simulink model "ctrl_DPAD_2"  (R2016b)
settings: Solver=ode3  StartTime=0.0  StopTime=inf  FixedStep=0.01  RelTol=1e-3  EnableMultiTasking=on
values from neighbouring files (symbols this model uses):
  C = [C1;C2;C3;C4;C5;C6]    [initfile.m]
  D = 3.0/100    (= 0.03)    [initfile.m]
  eps_c = 5    [initfile.m]
  epsilon = 0.5    [initfile.m]
  hd = c2d(H1,0.01,'foh')    [initfile.m]
  hd2 = c2d(H2,0.01,'zoh')    [initfile.m]
  I_s = 25000 /747225    (= 0.0334571246947)    [initfile.m]
  k_cc = 1    [initfile.m]
  K_omega = 0.3    [initfile.m]
  K_q1f = 0.0113    [initfile.m]
  K_q1r = K_q1f    (= 0.0113)    [initfile.m]
  K_q2f = 0.0117    [initfile.m]
  K_q2r = K_q2f    (= 0.0117)    [initfile.m]
  K_q3f = 0.0113    [initfile.m]
  K_q3r = K_q3f    (= 0.0113)    [initfile.m]
  K_q4f = 0.0169    [initfile.m]
  K_q4r = K_q4f    (= 0.0169)    [initfile.m]
  K_q5f = 0.0144    [initfile.m]
  K_q5r = K_q5f    (= 0.0144)    [initfile.m]
  K_q6f = 0.0168    [initfile.m]
  K_q6r = K_q6f    (= 0.0168)    [initfile.m]
  K_T1f = 0.3763    [initfile.m]
  K_T1r = K_T1f    (= 0.3763)    [initfile.m]
  K_T2f = 0.3901    [initfile.m]
  K_T2r = K_T2f    (= 0.3901)    [initfile.m]
  K_T3f = 0.3776    [initfile.m]
  K_T3r = K_T3f    (= 0.3776)    [initfile.m]
  K_T4f = 0.5641    [initfile.m]
  K_T4r = K_T4f    (= 0.5641)    [initfile.m]
  K_T5f = 0.4799    [initfile.m]
  K_T5r = K_T5f    (= 0.4799)    [initfile.m]
  K_T6f = 0.5588    [initfile.m]
  K_T6r = K_T6f    (= 0.5588)    [initfile.m]
  Kp = 3.3    [initfile.m]
  Max_Acceleration = 5    [initfile.m]
  Max_rotation = 12*sqrt(lambda)    [initfile.m]
  Max_thrust = 1.5    [initfile.m]
  Min_thrust = -0.8    [initfile.m]
  n_c = 5    [initfile.m]
  n_max = 152    [initfile.m]
  p_cc = 0.5    [initfile.m]
  pwm_thr1_backward = coeffvalues(ForceToPWM)    [initfile.m]
  pwm_thr1_forward = coeffvalues(ForceToPWM)    [initfile.m]
  pwm_thr2_backward = coeffvalues(ForceToPWM)    [initfile.m]
  pwm_thr2_forward = coeffvalues(ForceToPWM)    [initfile.m]
  pwm_thr3_backward = coeffvalues(ForceToPWM)    [initfile.m]
  pwm_thr3_forward = coeffvalues(ForceToPWM)    [initfile.m]
  pwm_thr4_backward = coeffvalues(ForceToPWM)    [initfile.m]
  pwm_thr4_forward = coeffvalues(ForceToPWM)    [initfile.m]
  pwm_thr5_backward = coeffvalues(ForceToPWM)    [initfile.m]
  pwm_thr5_forward = coeffvalues(ForceToPWM)    [initfile.m]
  pwm_thr6_backward = coeffvalues(ForceToPWM)    [initfile.m]
  pwm_thr6_forward = coeffvalues(ForceToPWM)    [initfile.m]
  Q_f0 = 0.3    [initfile.m]
  r_cc = 4    [initfile.m]
  Rho = Rho_m    (= 1000)    [initfile.m]
undefined symbols (not defined in the file or in its folder): DiscIntNeverNeededParam, Q_max, Thruster
libraries: marine_gnc x8, simulink x6, simulink_extras x3
(part 5 of 5)

== matlab function ctrl_DPAD_2/Thrust allocation/MATLAB Function ==
  data: u input; sys output; ThrusterPosX input; ThrusterPosY input; C input
function sys = fcn(u,ThrusterPosX,ThrusterPosY,C)
% Complete system goes here!
Alpha1 = zeros(1,6);    % Allocating dimensions for faster computing
% Parameters thrusters
tc =  [u(1),u(2),u(3)]'; 
alpha = [u(4),u(5),u(6),u(7),u(8),u(9)]';

% Constraints for Thruster-Thruster interaction. Can be seen in "Initfile"
% how they are found
C1 = C(1,:);
C2 = C(2,:);
C3 = C(3,:);
C4 = C(4,:);
C5 = C(5,:);
C6 = C(6,:);

K = ones(1,6);

K = ones(1,6);

if alpha(1) < C1(1)-0.1  && alpha(1) > C1(2)+0.1 || alpha(1) > C1(3)+0.1 && alpha(1) < C1(4)-0.1
    K(1) = 0;
else 
    K(1) = K(1);
end

if alpha(2) > C2(1)-0.1  && alpha(2) < C2(2)+0.1 || alpha(2) > C2(3)-0.1 && alpha(2) < C2(4)+0.1
    K(2) = 0;
else 
    K(2) = K(2);
end

if alpha(3) < C3(1)+0.1  && alpha(3) > C3(2)-0.1 || alpha(3) < C3(3)+0.1 && alpha(3) > C3(4)-0.1
    K(3) = 0;
else 
    K(3) = K(3);
end

if alpha(4) > C4(1)+0.1  && alpha(4) < C4(2)-0.1 || alpha(4) < C4(3)-0.1 && alpha(4) > C4(4)+0.1
    K(4) = 0;
else 
    K(4) = K(4);
end

if alpha(5) < C5(1)-0.1  && alpha(5) > C5(2)+0.1 || alpha(5) < C5(3)-0.1 && alpha(5) > C5(4)+0.1
    K(5) = 0;
else 
    K(5) = K(5);
end

if alpha(6) > C6(1)+0.1  && alpha(6) < C6(2)-0.1 || alpha(6) > C6(3)+0.1 && alpha(6) < C6(4)-0.1
    K(6) = 0;
else 
    K(6) = K(6);
end

epsilon = u(10);

n_t = length(ThrusterPosX); % number of thrusters
B_surge = zeros(n_t,1); % Shells for faster computing
B_sway = zeros(n_t,1);  % Shells for faster computing
B_yaw = zeros(n_t,1);   % Shells for faster computing

for i = 1:1:n_t
  B_surge(i) = cosd(alpha(i));     %Thrust in x-direction for cartesian
  B_sway(i) = sind(alpha(i));      %Thrust in y-direction for cartesian
  B_yaw(i) = (sind(alpha(i))*ThrusterPosX(i) - cosd(alpha(i))*ThrusterPosY(i));
end


B = [B_surge,B_sway,B_yaw]';
B = B*diag(K); 
[U_singular,S_singular,V_singular] = svd(B,'econ');
S_singular_cross = 1./S_singular;
S_singular_cross(~isfinite(S_singular_cross))=0;
 if (S_singular_cross(3,3)>10*S_singular_cross(2,2)) 
     S_singular_cross(3,3)=0;
 end
 
u_optimized = V_singular*S_singular_cross*U_singular';

u_d = u_optimized*tc;          % Optimized Thrust



Te = [1 0 1 0 1 0 1 0 1 0 1 0;
      0 1 0 1 0 1 0 1 0 1 0 1;
      ThrusterPosY(1) ThrusterPosX(1) ThrusterPosY(2) ThrusterPosX(2) ThrusterPosY(3) ThrusterPosX(3) ...
      ThrusterPosY(4) ThrusterPosX(4) ThrusterPosY(5) ThrusterPosX(5) ThrusterPosY(6) ThrusterPosX(6)];

[U_singular,S_singular,V_singular] = svd(Te,'econ');
S_singular_cross = 1./S_singular;
S_singular_cross(~isfinite(S_singular_cross))=0;
 if (S_singular_cross(3,3)>2*S_singular_cross(2,2)) 
     S_singular_cross(3,3)=0;
 end
T0 = V_singular*S_singular_cross*U_singular'*tc;

alpha1 = [atan2d(T0(2),T0(1)) atan2d(T0(4),T0(3)) atan2d(T0(6),T0(5)) atan2d(T0(8),T0(7)) atan2d(T0(10),T0(9)) atan2d(T0(12),T0(11))];


%% Constraints
% Thruster 1 OK
%C1 = [151 130 -151 -130 ];
if alpha1(1) < C1(1)  && alpha1(1) > C1(2) && u_d(1) > 0 || alpha1(1) < C1(1)  && alpha1(1) > C1(2) && u_d(1) < 0
    c1 = [C1(1) C1(2)];
    [C_1,alpha_new1] = min(abs(c1-alpha1(1)));
    Alpha1(1) = c1(alpha_new1);
elseif alpha1(1) > C1(3) && alpha1(1) < C1(4) && u_d(1) > 0 || alpha1(1) > C1(3) && alpha1(1) < C1(4) && u_d(1) < 0
    c1 = [C1(3) C1(4)];
    [C_1,alpha_new1] = min(abs(c1-alpha1(1)));
    Alpha1(1) = c1(alpha_new1);
else 
    Alpha1(1) = alpha1(1);
end
if alpha(1) < C1(1)-0.1  && alpha(1) > C1(2)+0.1 || alpha(1) > C1(3)+0.1 && alpha(1) < C1(4)-0.1
    u_d(1) = 0;
else 
    u_d(1) = u_d(1);
end

% Thruster 2 
%C2 = [-99.85 -80.15 -50 -29];
if alpha1(2) < C2(1)  && alpha1(2) > C2(2) && u_d(2) > 0 || alpha1(2) < C2(1)  && alpha1(2) > C2(2) && u_d(2) < 0 
    c2 = [C2(1) C2(2)];
    [C_2,alpha_new2] = min(abs(c2-alpha1(2)));
    Alpha1(2) = c2(alpha_new2);
elseif alpha1(2) < C2(3) && alpha1(2) > C2(4) && u_d(2) > 0 || alpha1(2) < C2(3) && alpha1(2) > C2(4) && u_d(2) < 0
    c2 = [C2(3) C2(4)];
    [C_2,alpha_new2] = min(abs(c2-alpha1(2)));
    Alpha1(2) = c2(alpha_new2);
else 
    Alpha1(2) = alpha1(2);
end
if alpha(2) < C2(1)-0.1  && alpha(2) > C2(2)+0.1 || alpha(2) < C2(3)-0.1 && alpha(2) > C2(4)+0.1
    u_d(2) = 0;
else 
    u_d(2) = u_d(2);
end

% Thruster 3 
% C3 = [99.85 80.15 50 29]; 

if alpha1(3) > C3(1)  && alpha1(3) < C3(2) && u_d(3) > 0 || alpha1(3) > C3(1)  && alpha1(3) < C3(2) && u_d(3) < 0
    c3 = [C3(1) C3(2)];
    [C_3,alpha_new3] = min(abs(c3-alpha1(3)));
    Alpha1(3) = c3(alpha_new3);
elseif alpha1(3) > C3(3) && alpha1(3) < C3(4) && u_d(3) > 0 || alpha1(3) > C3(3) && alpha1(3) < C3(4) && u_d(3) < 0 
    c3 = [C3(3) C3(4)];
    [C_3,alpha_new3] = min(abs(c3-alpha1(3)));
    Alpha1(3) = c3(alpha_new3);
else 
    Alpha1(3) = alpha1(3);
end
if alpha(3) > C3(1)+0.1  && alpha(3) < C3(2)-0.1 || alpha(3) > C3(3)+0.1 && alpha(3) < C3(4)-0.1
    u_d(3) = 0;
else 
    u_d(3) = u_d(3);
end

% Thruster 4 OK
%C4 = [-52.8 -34.2 52.8 34.2]; 
if alpha1(4) > C4(1)  && alpha1(4) < C4(2) && u_d(4) > 0 || alpha1(4) > C4(1)  && alpha1(4) < C4(2) && u_d(4) < 0
    c4 = [C4(1) C4(2)];
    [C_4,alpha_new4] = min(abs(c4-alpha1(4)));
    Alpha1(4) = c4(alpha_new4);
elseif alpha1(4) < C4(3) && alpha1(4) > C4(4) && u_d(4) > 0 || alpha1(4) < C4(3) && alpha1(4) > C4(4) && u_d(4) < 0 
    c4 = [C4(3) C4(4)];
    [C_4,alpha_new4] = min(abs(c4-alpha1(4)));
    Alpha1(4) = c4(alpha_new4);
else 
    Alpha1(4) = alpha1(4);
end
if alpha(4) > C4(1)+0.1  && alpha(4) < C4(2)-0.1 || alpha(4) < C4(3)-0.1 && alpha(4) > C4(4)+0.1
    u_d(4) = 0;
else 
    u_d(4) = u_d(4);
end

% Thruster 5
%C5 = [-98.25 -81.75 -145.8 -127.2];
if alpha1(5) < C5(1)  && alpha1(5) > C5(2) && u_d(5) > 0 || alpha1(5) < C5(1)  && alpha1(5) > C5(2) && u_d(5) < 0
    c5 = [C5(1) C5(2)];
    [C_5,alpha_new5] = min(abs(c5-alpha1(5)));
    Alpha1(5) = c5(alpha_new5);
elseif alpha1(5) < C5(3) && alpha1(5) > C5(4) && u_d(5) > 0  || alpha1(5) < C5(3) && alpha1(5) > C5(4) && u_d(5) < 0
    c5 = [C5(3) C5(4)];
    [C_5,alpha_new5] = min(abs(c5-alpha1(5)));
    Alpha1(5) = c5(alpha_new5);
else 
    Alpha1(5) = alpha1(5);
end
if alpha(5) < C5(1)-0.1  && alpha(5) > C5(2)+0.1 || alpha(5) < C5(3)-0.1 && alpha(5) > C5(4)+0.1
    u_d(5) = 0;
else 
    u_d(5) = u_d(5);
end

% Thruster 6
%C6 = [98.75 81.75 145.8 127.2];
if alpha1(6) > C6(1)  && alpha1(6) < C6(2) && u_d(6) > 0 || alpha1(6) > C6(1)  && alpha1(6) < C6(2) && u_d(6) < 0
    c6 = [C6(1) C6(2)];
    [C_6,alpha_new6] = min(abs(c6-alpha1(6)));
    Alpha1(6) = c6(alpha_new6);
elseif alpha1(6) > C6(3) && alpha1(6) < C6(4) && u_d(6) > 0 || alpha1(6) > C6(3) && alpha1(6) < C6(4) && u_d(6) < 0
    c6 = [C6(3) C6(4)];
    [C_6,alpha_new6] = min(abs(c6-alpha1(6)));
    Alpha1(6) = c6(alpha_new6);
else 
    Alpha1(6) = alpha1(6);
end
if alpha(6) > C6(1)+0.1  && alpha(6) < C6(2)-0.1 || alpha(6) > C6(3)+0.1 && alpha(6) < C6(4)-0.1
    u_d(6) = 0;
else 
    u_d(6) = u_d(6);
end

% Thruster 2&3 
if Alpha1(2) == C2(2)
    Alpha1(3) = alpha1(2) - (C2(2) - alpha1(2));
elseif Alpha1(2) == C2(1)
    Alpha1(3) = alpha1(2) - (C2(1) - alpha1(2));
elseif Alpha1(2) == C2(3)
    Alpha1(3) = alpha1(2) - (C2(3) - alpha1(2));
elseif Alpha1(2) == C2(4)
    Alpha1(3) = alpha1(2) - (C2(4) - alpha1(2));
    
elseif Alpha1(3) == C3(2)
    Alpha1(2) = alpha1(3) - (C3(2) - alpha1(3));
elseif Alpha1(3) == C3(1)
    Alpha1(2) = alpha1(3) - (C3(1) - alpha1(3));
elseif Alpha1(3) == C3(3)
    Alpha1(2) = alpha1(3) - (C3(3) - alpha1(3));
elseif Alpha1(3) == C3(4)
    Alpha1(2) = alpha1(3) - (C3(4) - alpha1(3));
end

% Thruster 5&6
if Alpha1(5) == C5(2)
    Alpha1(6) = alpha1(5) - (C5(2) - alpha1(5));
elseif Alpha1(5) == C5(1)
    Alpha1(6) = alpha1(5) - (C5(1) - alpha1(5));
elseif Alpha1(5) == C5(3)
    Alpha1(6) = alpha1(5) - (C5(3) - alpha1(5));
elseif Alpha1(5) == C5(4)
    Alpha1(6) = alpha1(5) - (C5(4) - alpha1(5));
    
elseif Alpha1(6) == C6(2)
    Alpha1(5) = alpha1(6) - (C6(2) - alpha1(6));
elseif Alpha1(6) == C6(1)
    Alpha1(5) = alpha1(6) - (C6(1) - alpha1(6));
elseif Alpha1(6) == C6(3)
    Alpha1(5) = alpha1(6) - (C6(3) - alpha1(6));
elseif Alpha1(6) == C6(4)
    Alpha1(5) = alpha1(6) - (C6(4) - alpha1(6));
end
% Thruster 4 & 1
if     Alpha1(4) == C4(2)
    Alpha1(1) = alpha1(4) - (C4(2) - alpha1(4));
elseif Alpha1(4) == C4(1)
    Alpha1(1) = alpha1(4) - (C4(1) - alpha1(4));
elseif Alpha1(4) == C4(3)
    Alpha1(1) = alpha1(4) - (C4(3) - alpha1(4));
elseif Alpha1(4) == C4(4)
    Alpha1(1) = alpha1(4) - (C4(4) - alpha1(4));
end

if     Alpha1(1) == C1(2)
    Alpha1(4) = alpha1(1) - (C1(2) - alpha1(1));
elseif Alpha1(1) == C1(1)
    Alpha1(4) = alpha1(1) - (C1(1) - alpha1(1));
elseif Alpha1(1) == C1(3)
    Alpha1(4) = alpha1(1) - (C1(3) - alpha1(1));
elseif Alpha1(1) == C1(4)
    Alpha1(4) = alpha1(1) - (C1(4) - alpha1(1));
end

Alpha1 = [Alpha1(1) Alpha1(2) Alpha1(3) Alpha1(4) Alpha1(5) Alpha1(6)]';    
Desired_thrust = [u_d(1) u_d(2) u_d(3) u_d(4) u_d(5) u_d(6)]';
alpha_desired = Alpha1;


% u_d = -Desired_thrust;
%% Update outputs
sys = [alpha_desired',u_d']';

== matlab function ctrl_DPAD_2/Thruster control /Thruster 1/Propeller Hydrodynamics/Actual Force and Torque ==
  data: Ta output; n input; Qa output; Kq input; Kt input; Ktr input; Kqr input; Rho input; D input; eps_c input; env input; Pa output
function [Ta,Qa,Pa]= ActualForces(n,Kq,Kt,Ktr,Kqr,Rho,D,eps_c,env)
%#codegen
lambda_c = 0.5+0.5*tanh(eps_c*n/5); % Smooth switching between positive and negative thrust. 5 makes switch happen between -5 and 5
K_TC = Kt*lambda_c+(1-lambda_c)*Ktr;
K_QC = Kq*lambda_c+(1-lambda_c)*Kqr;

Ta = sign(n)*K_TC*Rho*(D^4)*n^2-env;
Qa = sign(n)*K_QC*Rho*(D^5)*n^2-env;
Pa = 2*pi*n*Qa;

== matlab function ctrl_DPAD_2/Thruster control /Thruster 1/Thruster control/MATLAB Function ==
  data: Td input; n_d output; K_t0 input; K_t0r input; rho input; D input; eps_c input; n_c input; n_r input; T_r output
function [n_d,T_r]  = ReferenceGenerator(Td,K_t0,K_t0r,rho,D,eps_c,n_c,n_r)
%#codegen


n_d = sign(Td)*sqrt((abs(Td))/(rho*D^4*K_t0));

lambda_c = 0.5+0.5*tanh(eps_c*n_d/5); % Smooth switching between positive and negative thrust. 5 makes switch happen between -5 and 5
K_TC = K_t0*lambda_c+(1-lambda_c)*K_t0r;

T_r = sign(n_r)*K_TC*rho*D^4*n_r^2;

== matlab function ctrl_DPAD_2/Thruster control /Thruster 1/Thruster control/Supervisor ==
  data: control input; input input; n input; u output
function u = fcn(control,input,n)
u = 1;
if control == 1
if input == 1
    u = 1;
elseif input == 2
    u = 2;
elseif input == 3 && n > 0 || input == 3 && n < 0
    u = 3;
elseif input == 4 || input == 3 && n == 0
    u = 4;
else 
    u = 5;
end
end

if control == 2
if input == 1
    u = 1;
elseif input == 2
    u = 2;
elseif input == 3 && n > 0 || input == 3 && n < 0
    u = 3;
elseif input == 4 || input == 3 && n == 0
    u = 4;
else 
    u = 5;
end
end

if control == 3
if input == 1
    u = 1;
elseif input == 2
    u = 2;
elseif input == 3 && n > 0 || input == 3 && n < 0
    u = 3;
elseif input == 4 || input == 3 && n == 0
    u = 4;
else 
    u = 5;
end
end

if control == 4
if input == 1
    u = 1;
elseif input == 2
    u = 2;
elseif input == 3 && n > 0 || input == 3 && n < 0
    u = 3;
elseif input == 4 || input == 3 && n == 0
    u = 4;
else 
    u = 5;
end
end

if control == 5
if input == 1
    u = 1;
elseif input == 2
    u = 2;
elseif input == 3 && n > 0 || input == 3 && n < 0
    u = 3;
elseif input == 4 || input == 3 && n == 0
    u = 4;
else 
    u = 5;
end
end

== matlab function ctrl_DPAD_2/Thruster control /Thruster 1/Thruster control/Core controller/Core controller: Torque,Power and Combined Torque//Power ==
  data: Qcq output; Qcp output; k_cc input; p_cc input; r_cc input; n input; Qcc output; K_t0 input; K_q0 input; D input; Tr input; rho input; eps_c input; K_t0r input; K_q0r input
function [Qcq,Qcp,Qcc]= CoreControl(k_cc,p_cc,r_cc,n,K_t0,K_q0,D,Tr,rho,eps_c,K_t0r,K_q0r)
%#codegen

lambda_c = 0.5+0.5*tanh(eps_c*n/5);
K_TC = K_t0*lambda_c+(1-lambda_c)*K_t0r;
K_QC = K_q0*lambda_c+(1-lambda_c)*K_q0r;
Qcq = (K_QC/K_TC)*D*Tr;
if n == 0
    Qcp = 0;
else
Qcp = sign(Tr)*K_QC*(abs(Tr)^(3/2))/(sqrt(rho)*D*K_TC^(3/2)*abs(n));
end
alpha_c = exp(-k_cc*abs(p_cc*n)^r_cc);

Qcc = alpha_c*Qcq + (1-alpha_c)*Qcp;

== matlab function ctrl_DPAD_2/Thruster control /Thrust and Shaft speed mapped to PWM/MATLAB Function2 ==
  data: Tc_in1 input; signal input; Tc_out output; Tc_in2 input
function Tc_out = fcn(Tc_in1,signal,Tc_in2)
%#codegen

if signal >= 0
    Tc_out = Tc_in1;
else %signal < 0
    Tc_out = Tc_in2;
end

== matlab function ctrl_DPAD_2/Thruster control /Thruster 2/Propeller Hydrodynamics/Actual Force and Torque ==
  data: Ta output; n input; Qa output; Kq input; Kt input; Ktr input; Kqr input; Rho input; D input; eps_c input; env input
function [Ta,Qa]= ActualForces(n,Kq,Kt,Ktr,Kqr,Rho,D,eps_c,env)
%#codegen
lambda_c = 0.5+0.5*tanh(eps_c*n/5); % Smooth switching between positive and negative thrust. 5 makes switch happen between -5 and 5
K_TC = Kt*lambda_c+(1-lambda_c)*Ktr;
K_QC = Kq*lambda_c+(1-lambda_c)*Kqr;

Ta = sign(n)*K_TC*Rho*(D^4)*n^2-env;
Qa = sign(n)*K_QC*Rho*(D^5)*n^2-env;

== matlab function ctrl_DPAD_2/Finding commanded forces in: [Surge,Sway,Yaw] ==
  data: thrust_actual input; commanded_tau output; alpha_actual input; PosX input; PosY input
function commanded_tau   = fcn(thrust_actual,alpha_actual,PosX,PosY)
%#codegen

Alpha_surge =[cosd(alpha_actual(1)) cosd(alpha_actual(2)) cosd(alpha_actual(3)) cosd(alpha_actual(4)) cosd(alpha_actual(5)) cosd(alpha_actual(6))];  
Alpha_sway = [sind(alpha_actual(1)) sind(alpha_actual(2)) sind(alpha_actual(3)) sind(alpha_actual(4)) sind(alpha_actual(5)) sind(alpha_actual(6))];
Alpha_yaw = [sind(alpha_actual(1))*PosX(1)-cosd(alpha_actual(1))*PosY(1) sind(alpha_actual(2))*PosX(2)-cosd(alpha_actual(2))*PosY(2) ...
             sind(alpha_actual(3))*PosX(3)-cosd(alpha_actual(3))*PosY(3) sind(alpha_actual(4))*PosX(4)-cosd(alpha_actual(4))*PosY(4) ...
             sind(alpha_actual(5))*PosX(5)-cosd(alpha_actual(5))*PosY(5) sind(alpha_actual(6))*PosX(6)-cosd(alpha_actual(6))*PosY(6)];

commanded_tau = [Alpha_surge;Alpha_sway;Alpha_yaw]*thrust_actual;

== matlab function ctrl_DPAD_2/Thrust allocation/angle between [-180 180] ==
  data: angle input; y output
function y = rad2pipi(angle)
% RAD2PIPI Converts an angle in rad to the interval (-pi pi]
%          Should be applied to all heading errors in a feedback control system
%          in order to avoid discontinuities.
%
% Author:     Roger Skjetne
% Date:       2003-09-05
% Revisions:  2004-09-02 Thor I. Fossen - replaced input argument x with angle
%             2005-01-05 Thor I. Fossen - ouput argument is set to y and not angle
%             2005-04-13 Roger Skjetne  - changed the function s in order
%                                         to account for correct mapping to
%                                         (-pi pi].
%
% ________________________________________________________________
%
% MSS GNC is a Matlab toolbox for guidance, navigation and control.
% The toolbox is part of the Marine Systems Simulator (MSS).
%
% Copyright (C) 2008 Thor I. Fossen and Tristan Perez
% 
% This program is free software: you can redistribute it and/or modify
% it under the terms of the GNU General Public License as published by
% the Free Software Foundation, either version 3 of the License, or
% (at your option) any later version.
% 
% This program is distributed in the hope that it will be useful, but
% WITHOUT ANY WARRANTY; without even the implied warranty of
% MERCHANTABILITY or FITNESS FOR A PARTICULAR PURPOSE.  See the 
% GNU General Public License for more details.
% 
% You should have received a copy of the GNU General Public License
% along with this program.  If not, see <http://www.gnu.org/licenses/>.
% 
% E-mail: contact@marinecontrol.org
% URL:    <http://www.marinecontrol.org>


% convert angle in rad to the interval <-pi pi> 
r = rem(angle+sign(angle)*pi,2*pi);
s = sign(sign(angle) + 2*(sign(abs(rem(angle+pi,2*pi)/(2*pi)))-1));
% s = sign(angle);

y = r - s*pi;

== matlab function ctrl_DPAD_2/Input1/Guidance gains/MATLAB Function ==
  data: u input; y output
function y = fcn(u)

y = diag(u);

== matlab function ctrl_DPAD_2/Input1/Guidance gains/MATLAB Function1 ==
  data: u input; y output
function y = fcn(u)

y = diag(u);

== matlab function ctrl_DPAD_2/Thruster control /Thrust and Shaft speed mapped to PWM/MATLAB Function3 ==
  data: Tc_in1 input; signal input; Tc_out output; Tc_in2 input
function Tc_out = fcn(Tc_in1,signal,Tc_in2)
%#codegen

if signal >= 0
    Tc_out = Tc_in1;
else %signal < 0
    Tc_out = Tc_in2;
end

== matlab function ctrl_DPAD_2/Thruster control /Thruster 2/Thruster control/Core controller/Core controller: Torque,Power and Combined Torque//Power ==
  data: Qcq output; Qcp output; k_cc input; p_cc input; r_cc input; n input; Qcc output; K_t0 input; K_q0 input; D input; Tr input; rho input; eps_c input; K_t0r input; K_q0r input
function [Qcq,Qcp,Qcc]= CoreControl(k_cc,p_cc,r_cc,n,K_t0,K_q0,D,Tr,rho,eps_c,K_t0r,K_q0r)
%#codegen

lambda_c = 0.5+0.5*tanh(eps_c*n/5);
K_TC = K_t0*lambda_c+(1-lambda_c)*K_t0r;
K_QC = K_q0*lambda_c+(1-lambda_c)*K_q0r;
Qcq = (K_QC/K_TC)*D*Tr;
if n == 0
    Qcp = 0;
else
Qcp = sign(Tr)*K_QC*(abs(Tr)^(3/2))/(sqrt(rho)*D*K_TC^(3/2)*abs(n));
end
alpha_c = exp(-k_cc*abs(p_cc*n)^r_cc);

Qcc = alpha_c*Qcq + (1-alpha_c)*Qcp;

== matlab function ctrl_DPAD_2/Thruster control /Thruster 2/Thruster control/MATLAB Function ==
  data: Td input; n_d output; K_t0 input; K_t0r input; rho input; D input; eps_c input; n_c input; n_r input; T_r output
function [n_d,T_r]  = ReferenceGenerator(Td,K_t0,K_t0r,rho,D,eps_c,n_c,n_r)
%#codegen


n_d = sign(Td)*sqrt((abs(Td))/(rho*D^4*K_t0));

lambda_c = 0.5+0.5*tanh(eps_c*n_d/5); % Smooth switching between positive and negative thrust
K_TC = K_t0*lambda_c+(1-lambda_c)*K_t0r;

T_r = sign(n_r)*K_TC*rho*D^4*n_r^2;

== matlab function ctrl_DPAD_2/Thruster control /Thruster 2/Thruster control/Supervisor ==
  data: control input; input input; n input; u output
function u = fcn(control,input,n)
u = 1;
if control == 1
if input == 1
    u = 1;
elseif input == 2
    u = 2;
elseif input == 3 && n > 0 || input == 3 && n < 0
    u = 3;
elseif input == 4 || input == 3 && n == 0
    u = 4;
else 
    u = 5;
end
end

if control == 2
if input == 1
    u = 1;
elseif input == 2
    u = 2;
elseif input == 3 && n > 0 || input == 3 && n < 0
    u = 3;
elseif input == 4 || input == 3 && n == 0
    u = 4;
else 
    u = 5;
end
end

if control == 3
if input == 1
    u = 1;
elseif input == 2
    u = 2;
elseif input == 3 && n > 0 || input == 3 && n < 0
    u = 3;
elseif input == 4 || input == 3 && n == 0
    u = 4;
else 
    u = 5;
end
end

if control == 4
if input == 1
    u = 1;
elseif input == 2
    u = 2;
elseif input == 3 && n > 0 || input == 3 && n < 0
    u = 3;
elseif input == 4 || input == 3 && n == 0
    u = 4;
else 
    u = 5;
end
end

if control == 5
if input == 1
    u = 1;
elseif input == 2
    u = 2;
elseif input == 3 && n > 0 || input == 3 && n < 0
    u = 3;
elseif input == 4 || input == 3 && n == 0
    u = 4;
else 
    u = 5;
end
end

== matlab function ctrl_DPAD_2/Thruster control /Thrust and Shaft speed mapped to PWM/MATLAB Function4 ==
  data: Tc_in1 input; signal input; Tc_out output; Tc_in2 input
function Tc_out = fcn(Tc_in1,signal,Tc_in2)
%#codegen

if signal >= 0
    Tc_out = Tc_in1;
else %signal < 0
    Tc_out = Tc_in2;
end

== matlab function ctrl_DPAD_2/Thruster control /Thruster 3/Propeller Hydrodynamics/Actual Force and Torque ==
  data: Ta output; n input; Qa output; Kq input; Kt input; Ktr input; Kqr input; Rho input; D input; eps_c input; env input
function [Ta,Qa]= ActualForces(n,Kq,Kt,Ktr,Kqr,Rho,D,eps_c,env)
%#codegen
lambda_c = 0.5+0.5*tanh(eps_c*n/5); % Smooth switching between positive and negative thrust. 5 makes switch happen between -5 and 5
K_TC = Kt*lambda_c+(1-lambda_c)*Ktr;
K_QC = Kq*lambda_c+(1-lambda_c)*Kqr;

Ta = sign(n)*K_TC*Rho*(D^4)*n^2-env;
Qa = sign(n)*K_QC*Rho*(D^5)*n^2-env;

== matlab function ctrl_DPAD_2/Input1/Observer Gains/MATLAB Function ==
  data: u input; y output
function y = fcn(u)

y = diag(u);

== matlab function ctrl_DPAD_2/Thruster control /Thrust and Shaft speed mapped to PWM/MATLAB Function5 ==
  data: Tc_in1 input; signal input; Tc_out output; Tc_in2 input
function Tc_out = fcn(Tc_in1,signal,Tc_in2)
%#codegen

if signal >= 0
    Tc_out = Tc_in1;
else %signal < 0
    Tc_out = Tc_in2;
end

== matlab function ctrl_DPAD_2/Thruster control /Thruster 3/Thruster control/Core controller/Core controller: Torque,Power and Combined Torque//Power ==
  data: Qcq output; Qcp output; k_cc input; p_cc input; r_cc input; n input; Qcc output; K_t0 input; K_q0 input; D input; Tr input; rho input; eps_c input; K_t0r input; K_q0r input
function [Qcq,Qcp,Qcc]= CoreControl(k_cc,p_cc,r_cc,n,K_t0,K_q0,D,Tr,rho,eps_c,K_t0r,K_q0r)
%#codegen

lambda_c = 0.5+0.5*tanh(eps_c*n/5);
K_TC = K_t0*lambda_c+(1-lambda_c)*K_t0r;
K_QC = K_q0*lambda_c+(1-lambda_c)*K_q0r;
Qcq = (K_QC/K_TC)*D*Tr;
if n == 0
    Qcp = 0;
else
Qcp = sign(Tr)*K_QC*(abs(Tr)^(3/2))/(sqrt(rho)*D*K_TC^(3/2)*abs(n));
end
alpha_c = exp(-k_cc*abs(p_cc*n)^r_cc);

Qcc = alpha_c*Qcq + (1-alpha_c)*Qcp;

== matlab function ctrl_DPAD_2/Thruster control /Thruster 3/Thruster control/MATLAB Function ==
  data: Td input; n_d output; K_t0 input; K_t0r input; rho input; D input; eps_c input; n_c input; n_r input; T_r output
function [n_d,T_r]  = ReferenceGenerator(Td,K_t0,K_t0r,rho,D,eps_c,n_c,n_r)
%#codegen


n_d = sign(Td)*sqrt((abs(Td))/(rho*D^4*K_t0));

lambda_c = 0.5+0.5*tanh(eps_c*n_d/5); % Smooth switching between positive and negative thrust
K_TC = K_t0*lambda_c+(1-lambda_c)*K_t0r;

T_r = sign(n_r)*K_TC*rho*D^4*n_r^2;

== matlab function ctrl_DPAD_2/Thruster control /Thrust and Shaft speed mapped to PWM/MATLAB Function ==
  data: input input; output output; control input; speedcontrol input
function output = fcn(input,control,speedcontrol)
%#codegen
if control == 1
output = [input(1) speedcontrol(1) input(3) speedcontrol(2) input(5) speedcontrol(3) input(7) speedcontrol(4) input(9) speedcontrol(5) input(11) speedcontrol(6)]';
%     output = [input(1) input(2) input(3) input(4) input(5) input(6) input(7) input(8) input(9) input(10) input(11) input(12)]';

else
    output = [input(1) input(2) input(3) input(4) input(5) input(6) input(7) input(8) input(9) input(10) input(11) input(12)]';

end

== matlab function ctrl_DPAD_2/Thruster control /Thrust and Shaft speed mapped to PWM/MATLAB Function6 ==
  data: Tc_in1 input; signal input; Tc_out output; Tc_in2 input
function Tc_out = fcn(Tc_in1,signal,Tc_in2)
%#codegen

if signal >= 0
    Tc_out = Tc_in1;
else %signal < 0
    Tc_out = Tc_in2;
end

== matlab function ctrl_DPAD_2/Input1/Observer Gains/MATLAB Function1 ==
  data: u input; y output
function y = fcn(u)

y = diag(u);

== matlab function ctrl_DPAD_2/Input1/Observer Gains/MATLAB Function2 ==
  data: u input; y output
function y = fcn(u)

y = diag(u);

== matlab function ctrl_DPAD_2/Thruster control /Thruster 3/Thruster control/Supervisor ==
  data: control input; input input; n input; u output
function u = fcn(control,input,n)
u = 1;
if control == 1
if input == 1
    u = 1;
elseif input == 2
    u = 2;
elseif input == 3 && n > 0 || input == 3 && n < 0
    u = 3;
elseif input == 4 || input == 3 && n == 0
    u = 4;
else 
    u = 5;
end
end

if control == 2
if input == 1
    u = 1;
elseif input == 2
    u = 2;
elseif input == 3 && n > 0 || input == 3 && n < 0
    u = 3;
elseif input == 4 || input == 3 && n == 0
    u = 4;
else 
    u = 5;
end
end

if control == 3
if input == 1
    u = 1;
elseif input == 2
    u = 2;
elseif input == 3 && n > 0 || input == 3 && n < 0
    u = 3;
elseif input == 4 || input == 3 && n == 0
    u = 4;
else 
    u = 5;
end
end

if control == 4
if input == 1
    u = 1;
elseif input == 2
    u = 2;
elseif input == 3 && n > 0 || input == 3 && n < 0
    u = 3;
elseif input == 4 || input == 3 && n == 0
    u = 4;
else 
    u = 5;
end
end

if control == 5
if input == 1
    u = 1;
elseif input == 2
    u = 2;
elseif input == 3 && n > 0 || input == 3 && n < 0
    u = 3;
elseif input == 4 || input == 3 && n == 0
    u = 4;
else 
    u = 5;
end
end

== matlab function ctrl_DPAD_2/Control/MATLAB Function ==
  data: K_p output; K_p1 input
function K_p = fcn(K_p1)
%#codegen

K_p = diag(K_p1);

== matlab function ctrl_DPAD_2/Thruster control /Thruster 4/Propeller Hydrodynamics/Actual Force and Torque ==
  data: Ta output; n input; Qa output; Kq input; Kt input; Ktr input; Kqr input; Rho input; D input; eps_c input; env input
function [Ta,Qa]= ActualForces(n,Kq,Kt,Ktr,Kqr,Rho,D,eps_c,env)
%#codegen
lambda_c = 0.5+0.5*tanh(eps_c*n/5); % Smooth switching between positive and negative thrust. 5 makes switch happen between -5 and 5
K_TC = Kt*lambda_c+(1-lambda_c)*Ktr;
K_QC = Kq*lambda_c+(1-lambda_c)*Kqr;

Ta = sign(n)*K_TC*Rho*(D^4)*n^2-env;
Qa = sign(n)*K_QC*Rho*(D^5)*n^2-env;

== matlab function ctrl_DPAD_2/Thruster control /Thruster 4/Thruster control/Core controller/Core controller: Torque,Power and Combined Torque//Power ==
  data: Qcq output; Qcp output; k_cc input; p_cc input; r_cc input; n input; Qcc output; K_t0 input; K_q0 input; D input; Tr input; rho input; eps_c input; K_t0r input; K_q0r input
function [Qcq,Qcp,Qcc]= CoreControl(k_cc,p_cc,r_cc,n,K_t0,K_q0,D,Tr,rho,eps_c,K_t0r,K_q0r)
%#codegen

lambda_c = 0.5+0.5*tanh(eps_c*n/5);
K_TC = K_t0*lambda_c+(1-lambda_c)*K_t0r;
K_QC = K_q0*lambda_c+(1-lambda_c)*K_q0r;
Qcq = (K_QC/K_TC)*D*Tr;
if n == 0
    Qcp = 0;
else
Qcp = sign(Tr)*K_QC*(abs(Tr)^(3/2))/(sqrt(rho)*D*K_TC^(3/2)*abs(n));
end
alpha_c = exp(-k_cc*abs(p_cc*n)^r_cc);

Qcc = alpha_c*Qcq + (1-alpha_c)*Qcp;

== matlab function ctrl_DPAD_2/Thruster control /Thruster 4/Thruster control/MATLAB Function ==
  data: Td input; n_d output; K_t0 input; K_t0r input; rho input; D input; eps_c input; n_c input; n_r input; T_r output
function [n_d,T_r]  = ReferenceGenerator(Td,K_t0,K_t0r,rho,D,eps_c,n_c,n_r)
%#codegen


n_d = sign(Td)*sqrt((abs(Td))/(rho*D^4*K_t0));

lambda_c = 0.5+0.5*tanh(eps_c*n_d/5); % Smooth switching between positive and negative thrust
K_TC = K_t0*lambda_c+(1-lambda_c)*K_t0r;

T_r = sign(n_r)*K_TC*rho*D^4*n_r^2;

== matlab function ctrl_DPAD_2/Thruster control /Thruster 4/Thruster control/Supervisor ==
  data: control input; input input; n input; u output
function u = fcn(control,input,n)
u = 1;
if control == 1
if input == 1
    u = 1;
elseif input == 2
    u = 2;
elseif input == 3 && n > 0 || input == 3 && n < 0
    u = 3;
elseif input == 4 || input == 3 && n == 0
    u = 4;
else 
    u = 5;
end
end

if control == 2
if input == 1
    u = 1;
elseif input == 2
    u = 2;
elseif input == 3 && n > 0 || input == 3 && n < 0
    u = 3;
elseif input == 4 || input == 3 && n == 0
    u = 4;
else 
    u = 5;
end
end

if control == 3
if input == 1
    u = 1;
elseif input == 2
    u = 2;
elseif input == 3 && n > 0 || input == 3 && n < 0
    u = 3;
elseif input == 4 || input == 3 && n == 0
    u = 4;
else 
    u = 5;
end
end

if control == 4
if input == 1
    u = 1;
elseif input == 2
    u = 2;
elseif input == 3 && n > 0 || input == 3 && n < 0
    u = 3;
elseif input == 4 || input == 3 && n == 0
    u = 4;
else 
    u = 5;
end
end

if control == 5
if input == 1
    u = 1;
elseif input == 2
    u = 2;
elseif input == 3 && n > 0 || input == 3 && n < 0
    u = 3;
elseif input == 4 || input == 3 && n == 0
    u = 4;
else 
    u = 5;
end
end

== matlab function ctrl_DPAD_2/Control/MATLAB Function1 ==
  data: K_p output; K_p1 input
function K_p = fcn(K_p1)
%#codegen

K_p = diag(K_p1);

== matlab function ctrl_DPAD_2/Thruster control /Thruster 5/Propeller Hydrodynamics/Actual Force and Torque ==
  data: Ta output; n input; Qa output; Kq input; Kt input; Ktr input; Kqr input; Rho input; D input; eps_c input; env input
function [Ta,Qa]= ActualForces(n,Kq,Kt,Ktr,Kqr,Rho,D,eps_c,env)
%#codegen
lambda_c = 0.5+0.5*tanh(eps_c*n/5); % Smooth switching between positive and negative thrust. 5 makes switch happen between -5 and 5
K_TC = Kt*lambda_c+(1-lambda_c)*Ktr;
K_QC = Kq*lambda_c+(1-lambda_c)*Kqr;

Ta = sign(n)*K_TC*Rho*(D^4)*n^2-env;
Qa = sign(n)*K_QC*Rho*(D^5)*n^2-env;

== matlab function ctrl_DPAD_2/Thruster control /Thruster 5/Thruster control/Core controller/Core controller: Torque,Power and Combined Torque//Power ==
  data: Qcq output; Qcp output; k_cc input; p_cc input; r_cc input; n input; Qcc output; K_t0 input; K_q0 input; D input; Tr input; rho input; eps_c input; K_t0r input; K_q0r input
function [Qcq,Qcp,Qcc]= CoreControl(k_cc,p_cc,r_cc,n,K_t0,K_q0,D,Tr,rho,eps_c,K_t0r,K_q0r)
%#codegen

lambda_c = 0.5+0.5*tanh(eps_c*n/5);
K_TC = K_t0*lambda_c+(1-lambda_c)*K_t0r;
K_QC = K_q0*lambda_c+(1-lambda_c)*K_q0r;
Qcq = (K_QC/K_TC)*D*Tr;
if n == 0
    Qcp = 0;
else
Qcp = sign(Tr)*K_QC*(abs(Tr)^(3/2))/(sqrt(rho)*D*K_TC^(3/2)*abs(n));
end
alpha_c = exp(-k_cc*abs(p_cc*n)^r_cc);

Qcc = alpha_c*Qcq + (1-alpha_c)*Qcp;

== matlab function ctrl_DPAD_2/Thruster control /Thruster 5/Thruster control/MATLAB Function ==
  data: Td input; n_d output; K_t0 input; K_t0r input; rho input; D input; eps_c input; n_c input; n_r input; T_r output
function [n_d,T_r]  = ReferenceGenerator(Td,K_t0,K_t0r,rho,D,eps_c,n_c,n_r)
%#codegen


n_d = sign(Td)*sqrt((abs(Td))/(rho*D^4*K_t0));

lambda_c = 0.5+0.5*tanh(eps_c*n_d/5); % Smooth switching between positive and negative thrust
K_TC = K_t0*lambda_c+(1-lambda_c)*K_t0r;

T_r = sign(n_r)*K_TC*rho*D^4*n_r^2;

== matlab function ctrl_DPAD_2/Thruster control /Thruster 5/Thruster control/Supervisor ==
  data: control input; input input; n input; u output
function u = fcn(control,input,n)
u = 1;
if control == 1
if input == 1
    u = 1;
elseif input == 2
    u = 2;
elseif input == 3 && n > 0 || input == 3 && n < 0
    u = 3;
elseif input == 4 || input == 3 && n == 0
    u = 4;
else 
    u = 5;
end
end

if control == 2
if input == 1
    u = 1;
elseif input == 2
    u = 2;
elseif input == 3 && n > 0 || input == 3 && n < 0
    u = 3;
elseif input == 4 || input == 3 && n == 0
    u = 4;
else 
    u = 5;
end
end

if control == 3
if input == 1
    u = 1;
elseif input == 2
    u = 2;
elseif input == 3 && n > 0 || input == 3 && n < 0
    u = 3;
elseif input == 4 || input == 3 && n == 0
    u = 4;
else 
    u = 5;
end
end

if control == 4
if input == 1
    u = 1;
elseif input == 2
    u = 2;
elseif input == 3 && n > 0 || input == 3 && n < 0
    u = 3;
elseif input == 4 || input == 3 && n == 0
    u = 4;
else 
    u = 5;
end
end

if control == 5
if input == 1
    u = 1;
elseif input == 2
    u = 2;
elseif input == 3 && n > 0 || input == 3 && n < 0
    u = 3;
elseif input == 4 || input == 3 && n == 0
    u = 4;
else 
    u = 5;
end
end

== matlab function ctrl_DPAD_2/Control/MATLAB Function4 ==
  data: Eta input; tau1 output; z_1 output; tau_L output; tau_U output; Chi_tilde output; nu input; Eta_t input; Eta_tdot input; Eta_tdotdot input; z_2 output; K_p input; K_d input
  function [ tau1,z_1,tau_L,tau_U,Chi_tilde,z_2] = Cascaded_feedback_controller_LP_LV(Eta,nu,Eta_t,Eta_tdot,Eta_tdotdot,K_p,K_d)
%  [ tau,theta ] = Adaptiv_controller(Eta,nu,nu_dot,phi,theta_t,Eta_d,Eta_dtheta,Eta_dtheta2,v_s,v_stheta,v_st,h)
%UNTITLED6 Summary of this function goes here Skjetne
%   Detailed explanation goes here
%kan være den må løses på en smartere måte
%include Model_c to path
%#codegen
persistent PHI OMEGA_N EPSI_RR EPSI_PHI RR PHIPHI p_r p_p S_old_RR S_old_PHI pp YY_r YY_phi


stored_data=20;
if (isempty(PHI)||isempty(OMEGA_N))
    PHI=zeros(8,1);
    OMEGA_N=zeros(3,1);
    PHIPHI=zeros(8,3*stored_data);
    RR=zeros(3,3*stored_data);
    EPSI_RR=zeros(3*stored_data,1);
    EPSI_PHI=zeros(3*stored_data,1);
    S_old_RR=0;
    S_old_PHI=0;
    p_r=1;
    p_p=1;
    pp=1;
    YY_r=zeros(3*stored_data,1);
    YY_phi=zeros(3*stored_data,1);
end

 m    = 127.92;%14.79;
 x_g  = 0;%0.0375;
 I_z  =  61.967;%1.7600;  
 
 X_ud  =    3.262; %-2.0;											% Table B.1
 Y_vd =     28.89;%-10.0;
 N_vd =    0.157;%-0.0;		% Table B.1
 Y_rd =    0.525;%  -0.0;
 N_rd =    13.98;%-1.0;		% Table B.1

    M_RB_c=[m     0      0;
          0     m      m*x_g;
          0     m*x_g  I_z];
    M_A_c=[-X_ud    0          0;
            0          -Y_vd  -Y_rd;
            0          -N_vd  -N_rd];     
    M_c=M_RB_c+M_A_c;
    
    %   
%% Damping coefficients
% Comments at the end of the lines indicate the old values used.
X_u		= -2.332;%-0.6555;		X_v		= 0;
X_uu 	= 0;%0.3545;		X_vv	= -2.443;
X_uuu 	= -8.557;%-3.787;		X_vvv	= 0;

						Y_v		= -4.673;%-1.33; 			Y_r		= -7.250; % Y_r
						Y_vv	= 0.3976;%-2.776;			Y_rr	= -3.450; % Y_rr
						Y_vvv	= 313.3;%-64.91;			Y_rrr	= 0;
				
                        Y_r		= 0;%-7.250; % Y_r
                        Y_rr	= 0;%-3.450; % Y_rr
                        Y_rrr	= 0;
                        
                        
						%Y_rv	= -0.805;			Y_vr	= -0.845; % Y_rv, Y_vr

						N_v		= 0;				%N_r		= -1.900; % N_r
						N_vv	= -0.2088;			%N_rr	= -0.750; % N_rr
						N_vvv	= 0;				%N_rrr	= 0;
						
                        N_r		= -0.01675;%-1.900; % N_r
                        N_rr	= -0.01148;%-0.750; % N_rr
                        N_rrr	= 0.0003578;%0;
						%N_rv	= 0.130;			N_vr	= 0.080; % N_rv, N_vr
    
    
    
R=Rot(Eta);

u   = nu(1);
v   = nu(2);
r   = nu(3);

d_11 = -X_u - X_uu*abs(u) - X_uuu*u^2;
d_22 = -Y_v - Y_vv*abs(v) - Y_vvv*v^2; %- Y_rv*abs(r);
d_33 = -N_r - N_rr*abs(r) - N_rrr*r^2; %- N_vr*abs(v); % using abs(r)

d_12 = 0;%-X_v - X_vv*v - X_vvv*v^2;
d_23 = -Y_r - Y_rr*abs(r) - Y_rrr*r^2;% - Y_vr*abs(v);
d_32 = -N_v - N_vv*abs(v) - N_vvv*v^2;% - N_rv*abs(r);

D    = [d_11 d_12 0
        0    d_22 d_23
        0    d_32 d_33];
  
%% controlsignaler
Eta_tilde=Eta-Eta_t;
Chi_tilde=Eta(3)-Eta_t(3);
Chi_tilde=mod(pi/2+Chi_tilde,pi)-pi/2; %%%%%%%%%%%%%%%%%%%%%%

%% New Controller
z_1=R'*(Eta_tilde);

Alpha_1=(-K_p*z_1+(R')*Eta_tdot);
z_2=nu-Alpha_1;

z_1_dot=S(nu)'*z_1-K_p*z_1+z_2;
Alpha_1dot=-K_p*z_1_dot+S(nu)'*R'*Eta_tdot + R'*Eta_tdotdot;

% TAU 
tau=C_c(nu)*nu+D*nu+M_c*Alpha_1dot-K_d*z_2;
tau1=tau;

%%
tau_L=-K_d*z_2+M_c*Alpha_1dot;
tau_U=C_c(nu)*nu+D*nu;

end

    function matrix=C_c(V) %%Coreolis matrix
    %#codegen
        matrix=C_RB_c(V)+C_A_c(V);
    end
      function matrix=C_RB_c(V)
      %#codegen
 m    = 127.92;%14.79;
 x_g  = 0;%0.0375;
 I_z  =  61.967;%1.7600;  
            u=V(1);
            v=V(2);
            r=V(3);
            matrix=[0        0       -m*(x_g*r+v);
                    0        0        m*u;
                    m*(x_g*r+v) -m*u    0]; 
      end
      function matrix=C_A_c(V)
      %#codegen
 X_ud  =    3.262; %-2.0;											% Table B.1
 Y_vd =     28.89;%-10.0;
 N_vd =    0.157;%-0.0;		% Table B.1
 Y_rd =    0.525;%  -0.0;
 N_rd =    13.98;%-1.0;		% Table B.1

            u=V(1);
            v=V(2);
            r=V(3);
        matrix=[0                                      0              Y_vd*v+0.5*(N_vd+Y_rd)*r;
               0                                       0             -X_ud*u;
               -Y_vd*v-0.5*(N_vd+Y_rd)*r         X_ud*u       0]; 
      end   
%{      
function [ d ] = G_d(nu)
      %#codegen
X_u		= -0.6555;
Y_v		= -1.33;
N_v		= 0;

    v=[nu(1) nu(2) 0]';

      D_L_uv=[-X_u    0  0 ;
            0     -Y_v 0;
            0     -N_v 0];
      d=(D_L_uv+D_NL_uv(v))*v;

end

function matrix = D_NL_uv(V)
      %#codegen


 
	
X_uu 	= 0.3545;		X_vv	= -2.443;
X_uuu 	= -3.787;	

			
Y_vv	= -2.776;			
Y_vvv	= -64.91;

N_vv	= -0.2088;	

    u=V(1);
    v=V(2);
    
     matrix=[-X_uu*abs(u)-X_uuu*u^2 0 0;
            0 -Y_vv*abs(v)-Y_vvv*v^2 0;
            0 -N_vv*abs(v) 0];
end
%}
function matrix=Rot(N)
      %#codegen

    yaw=N(3);
    matrix=[cos(yaw) -sin(yaw) 0;
            sin(yaw)  cos(yaw) 0;
            0         0        1]; 
end
%{
function R_d = Rot_dot(nu,eta)
%% takes in the nu vector 
      %#codegen


R_d=S([0 0 nu(3)])*Rot([0 0 eta(3)]);

end
%}
function [ s ] = S(r)
%UNTITLED2 Summary of this function goes here
%   Detailed explanation goes here
      %#codegen

s=[0 -r(3) r(2);
   r(3) 0 -r(1);
   -r(2) r(1) 0];

end
%{
function [ phi ] = Phi( nu )
%UNTITLED3 Summary of this function goes here
%   Detailed explanation goes here
      %#codegen

v=nu(2);
IvI=abs(v);
r=nu(3);
IrI=abs(r);

phi=[0 0 0 0 0 0 0 0;
     -IrI*v -r -IvI*r -IrI*r 0 0 0 0;
     0 0 0 0 -IrI*v -r -IvI*r -IrI*r];

end
%}

== matlab function ctrl_DPAD_2/Thruster control /Thruster 6/Propeller Hydrodynamics/Actual Force and Torque ==
  data: Ta output; n input; Qa output; Kq input; Kt input; Ktr input; Kqr input; Rho input; D input; eps_c input; env input
function [Ta,Qa]= ActualForces(n,Kq,Kt,Ktr,Kqr,Rho,D,eps_c,env)
%#codegen
lambda_c = 0.5+0.5*tanh(eps_c*n/5); % Smooth switching between positive and negative thrust. 5 makes switch happen between -5 and 5
K_TC = Kt*lambda_c+(1-lambda_c)*Ktr;
K_QC = Kq*lambda_c+(1-lambda_c)*Kqr;

Ta = sign(n)*K_TC*Rho*(D^4)*n^2-env;
Qa = sign(n)*K_QC*Rho*(D^5)*n^2-env;

== matlab function ctrl_DPAD_2/Thruster control /Thruster 6/Thruster control/Core controller/Core controller: Torque,Power and Combined Torque//Power ==
  data: Qcq output; Qcp output; k_cc input; p_cc input; r_cc input; n input; Qcc output; K_t0 input; K_q0 input; D input; Tr input; rho input; eps_c input; K_t0r input; K_q0r input
function [Qcq,Qcp,Qcc]= CoreControl(k_cc,p_cc,r_cc,n,K_t0,K_q0,D,Tr,rho,eps_c,K_t0r,K_q0r)
%#codegen

lambda_c = 0.5+0.5*tanh(eps_c*n/5);
K_TC = K_t0*lambda_c+(1-lambda_c)*K_t0r;
K_QC = K_q0*lambda_c+(1-lambda_c)*K_q0r;
Qcq = (K_QC/K_TC)*D*Tr;
if n == 0
    Qcp = 0;
else
Qcp = sign(Tr)*K_QC*(abs(Tr)^(3/2))/(sqrt(rho)*D*K_TC^(3/2)*abs(n));
end
alpha_c = exp(-k_cc*abs(p_cc*n)^r_cc);

Qcc = alpha_c*Qcq + (1-alpha_c)*Qcp;

== matlab function ctrl_DPAD_2/Thruster control /Thruster 6/Thruster control/MATLAB Function ==
  data: Td input; n_d output; K_t0 input; K_t0r input; rho input; D input; eps_c input; n_c input; n_r input; T_r output
function [n_d,T_r]  = ReferenceGenerator(Td,K_t0,K_t0r,rho,D,eps_c,n_c,n_r)
%#codegen


n_d = sign(Td)*sqrt((abs(Td))/(rho*D^4*K_t0));

lambda_c = 0.5+0.5*tanh(eps_c*n_d/27); % Smooth switching between positive and negative thrust
K_TC = K_t0*lambda_c+(1-lambda_c)*K_t0r;

T_r = sign(n_r)*K_TC*rho*D^4*n_r^2;

== matlab function ctrl_DPAD_2/Thruster control /Thruster 6/Thruster control/Supervisor ==
  data: control input; input input; n input; u output
function u = fcn(control,input,n)
u = 1;
if control == 1
if input == 1
    u = 1;
elseif input == 2
    u = 2;
elseif input == 3 && n > 0 || input == 3 && n < 0
    u = 3;
elseif input == 4 || input == 3 && n == 0
    u = 4;
else 
    u = 5;
end
end

if control == 2
if input == 1
    u = 1;
elseif input == 2
    u = 2;
elseif input == 3 && n > 0 || input == 3 && n < 0
    u = 3;
elseif input == 4 || input == 3 && n == 0
    u = 4;
else 
    u = 5;
end
end

if control == 3
if input == 1
    u = 1;
elseif input == 2
    u = 2;
elseif input == 3 && n > 0 || input == 3 && n < 0
    u = 3;
elseif input == 4 || input == 3 && n == 0
    u = 4;
else 
    u = 5;
end
end

if control == 4
if input == 1
    u = 1;
elseif input == 2
    u = 2;
elseif input == 3 && n > 0 || input == 3 && n < 0
    u = 3;
elseif input == 4 || input == 3 && n == 0
    u = 4;
else 
    u = 5;
end
end

if control == 5
if input == 1
    u = 1;
elseif input == 2
    u = 2;
elseif input == 3 && n > 0 || input == 3 && n < 0
    u = 3;
elseif input == 4 || input == 3 && n == 0
    u = 4;
else 
    u = 5;
end
end

== matlab function ctrl_DPAD_2/Guidance/Reference model/w_d*w_d ==
  data: w_d input; y output
function y = fcn(w_d)
%#codegen

y = w_d*w_d;

== matlab function ctrl_DPAD_2/Guidance/Reference model/w_d*w_d1 ==
  data: w_d input; y output; zeta input
function y = fcn(w_d,zeta)
%#codegen

y = 2*zeta*w_d;

== matlab function ctrl_DPAD_2/Guidance/Reference model/w_d^-2 ==
  data: w_d input; y output
function y = fcn(w_d)
%#codegen

y = w_d^-2;

== matlab function ctrl_DPAD_2/Guidance/Reference model/w_d^3 ==
  data: w_d input; y output
function y = fcn(w_d)
%#codegen

y = w_d^3;

== matlab function ctrl_DPAD_2/Nonlinear Passisve Observer/C(nu)*nu ==
  data: nu_hat input; C_nl output
function C_nl = fcn(nu_hat)
%#codegen
u = nu_hat(1);
v = nu_hat(2);
r = nu_hat(3);

%% MATRICES
m    = 127.92;   x_g = 0; %0.0432;

%% Added mass
X_ud  =   3.262;	Y_vd =      28.89;		Y_rd =      0.525;

%% Correolis matrix
c_13 = -(m-Y_vd)*v-(m*x_g-Y_rd)*r;
c_23 = (m-X_ud)*u;

C    = [0     0     c_13
        0     0     c_23
        -c_13 -c_23 0   ];

    
C_NL = C;

C_nl =C_NL*nu_hat;

== matlab function ctrl_DPAD_2/Nonlinear Passisve Observer/D(nu)*nu ==
  data: nu_hat input; D_nl output
function D_nl = fcn(nu_hat)
%#codegen
u = nu_hat(1);
v = nu_hat(2);
r = nu_hat(3);

%% DAMPING 

% Surge:
% Based on fitting of towing data from -0.8 < u < 0.8 m/s
X_u     = -2.332;
X_uu	=  0;
X_uuu	= -8.557;

% Sway:
% Based on fitting of towing data from -0.45 < u < 0.45 m/s
Y_v 	= -4.673;
Y_vv	=  0.3976;
Y_vvv	= -313.3;

% Yaw:
% Based on fitting of towing data from -8 < u < 8 deg/s
% The fitting range is limited. Towing should be performed for higher
% velocities.
N_r		= -0.01675;
N_rr	= -0.01148;
N_rrr	= -0.0003578;

% Y_vvv og N_rrr er fra curvefitting uten minus, men ser ut til å fungere
% med minus. 
                           N_v		= 0;                Y_r	    =  -7.250; 
                           N_vv	    = -0.2088;          Y_rr	=  -3.450;
                           N_vvv	= 0;                Y_rrr	=  0;
						
						   Y_rv	    = -0.805;			Y_vr	=  -0.845; 

						   N_rv	    = 0.08;             N_vr	= 0.08;
                           
%% Assembly of the damping matrix
d_11 = X_u + X_uu*abs(u) + X_uuu*u^2;
d_22 = Y_v + Y_vv*abs(v) + Y_vvv*v^2;
d_33 = N_r + N_rr*abs(r) + N_rrr*r^2;

d_23 = 0; % Y_r + Y_rr*abs(r) + Y_rrr*r^2 + Y_vr*abs(v); Not verified, temporarily disabled
d_32 = 0; % N_v + N_vv*abs(v) + N_vvv*v^2 + N_rv*abs(r); Not verified, temporarily disabled

D    = - [d_11 0    0
          0    d_22 d_23
          0    d_32 d_33];


D_NL = D;

D_nl =D_NL*nu_hat;
